simulink model "modelitos"  (R2018a)
settings: Solver=ode4  StartTime=0.0  StopTime=1000  FixedStep=0.002  RelTol=1e-3
libraries: simulink x1
settings Model: Creator=heitor  LastModifiedBy=heitor

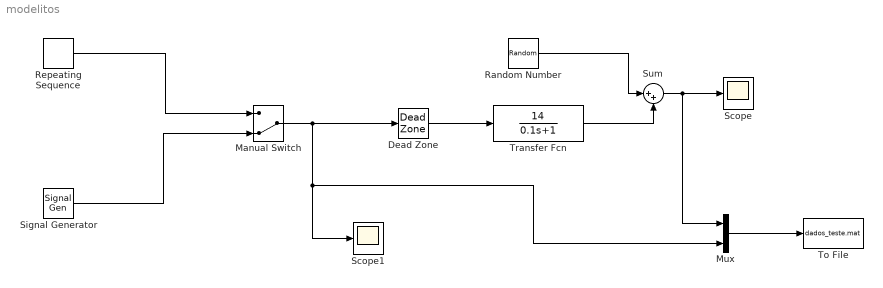
== system modelitos ==
  Dead Zone : DeadZone  LowerValue=-1.2  SaturateOnIntegerOverflow=on
  Manual Switch : ManualSwitch  CurrentSetting=0
  Mux : Mux  Inputs=2
  Random Number : RandomNumber  SampleTime=0.002
  Repeating Sequence : simulink/Sources/Repeating Sequence  rep_seq_t=[0 1 2 3 4]*5  rep_seq_y=[0 1 0 -1 0]*3
  Scope : Scope
  Scope1 : Scope
  Signal Generator : SignalGenerator  WaveForm=square  Amplitude=20  Units=rad/sec
  Sum : Sum  Inputs=|++
  To File : ToFile  Filename=dados_teste.mat  MatrixName=dados
  Transfer Fcn : TransferFcn  Numerator=14  Denominator=[0.1 1]
  wires:
  Mux/1 -> To File/1
  Dead Zone/1 -> Transfer Fcn/1
  Transfer Fcn/1 -> Sum/2
  Sum/1 -> Mux/1, Scope/1
  Random Number/1 -> Sum/1
  Repeating Sequence/1 -> Manual Switch/1
  Manual Switch/1 -> Mux/2, Scope1/1, Dead Zone/1
  Signal Generator/1 -> Manual Switch/2
